simulink model "snb_bc"  (R2012b)
settings: Solver=FixedStepDiscrete  SolverMode=SingleTasking  StartTime=0.0  StopTime=10000  RelTol=1e-3
undefined symbols (not defined in the file): Down, pfb_coeff_gen_calc, Up
libraries: xbsIndex_r4 x19640, casper_library_misc x44, casper_library_delays x18, casper_library_communications x8, xps_library x3
(part 12 of 163)

== system snb_bc/gbe_status ==
  out_gbe0_linkup : Inport
  out_gbe1_linkup : Inport  Port=2
  out_gbe2_linkup : Inport  Port=3
  out_gbe3_linkup : Inport  Port=4
  assert_gbe0_linkup : xbsIndex_r4/Assert  assert_type=on  type_source=Explicitly  gui_display_data_type=Boolean  arith_type=Boolean  n_bits=1  bin_pt=0  preci_type=Single  exp_width=8  frac_width=24  assert_rate=off  rate_source=Explicitly  period=1  output_port=on  block_type=assert
  assert_gbe1_linkup : xbsIndex_r4/Assert  assert_type=on  type_source=Explicitly  gui_display_data_type=Boolean  arith_type=Boolean  n_bits=1  bin_pt=0  preci_type=Single  exp_width=8  frac_width=24  assert_rate=off  rate_source=Explicitly  period=1  output_port=on  block_type=assert
  assert_gbe2_linkup : xbsIndex_r4/Assert  assert_type=on  type_source=Explicitly  gui_display_data_type=Boolean  arith_type=Boolean  n_bits=1  bin_pt=0  preci_type=Single  exp_width=8  frac_width=24  assert_rate=off  rate_source=Explicitly  period=1  output_port=on  block_type=assert
  assert_gbe3_linkup : xbsIndex_r4/Assert  assert_type=on  type_source=Explicitly  gui_display_data_type=Boolean  arith_type=Boolean  n_bits=1  bin_pt=0  preci_type=Single  exp_width=8  frac_width=24  assert_rate=off  rate_source=Explicitly  period=1  output_port=on  block_type=assert
  cast_gw : xbsIndex_r4/Convert  gui_display_data_type=Fixed-point  arith_type=Unsigned  n_bits=32  bin_pt=0  float_type=Single  exp_bits=8  fraction_bits=24  quantization=Truncate  overflow=Wrap  en=off  latency=0  dbl_ovrd=off  pipeline=off  block_type=convert
  concatenate : xbsIndex_r4/Concat  num_inputs=4  dbl_ovrd=off  block_type=concat
  io_delay : xbsIndex_r4/Delay  rst=off  infoeditControl=Selection of Reset will increase slice count due to use of real FFs and instead of SRLs  en=off  latency=0  dbl_ovrd=off  reg_retiming=on  block_type=delay
  reint{1..4} (4 alike) : xbsIndex_r4/Reinterpret  force_arith_type=on  arith_type=Unsigned  force_bin_pt=on  bin_pt=0  block_type=reinterpret
  sim_out : Terminator
  snb_bc_gbe_status_user_data_in : xbsIndex_r4/Gateway Out  inherit_from_input=off  hdl_port=on  timing_constraint=None  locs_specified=off  LOCs={}  UseAsDAC=off  DACChannel='1'  block_type=gatewayout
  wires:
  concatenate/1 -> io_delay/1
  io_delay/1 -> cast_gw/1
  cast_gw/1 -> snb_bc_gbe_status_user_data_in/1
  snb_bc_gbe_status_user_data_in/1 -> sim_out/1
  out_gbe0_linkup/1 -> assert_gbe0_linkup/1
  assert_gbe0_linkup/1 -> reint1/1
  reint1/1 -> concatenate/1
  out_gbe1_linkup/1 -> assert_gbe1_linkup/1
  assert_gbe1_linkup/1 -> reint2/1
  reint2/1 -> concatenate/2
  out_gbe2_linkup/1 -> assert_gbe2_linkup/1
  assert_gbe2_linkup/1 -> reint3/1
  reint3/1 -> concatenate/3
  out_gbe3_linkup/1 -> assert_gbe3_linkup/1
  assert_gbe3_linkup/1 -> reint4/1
  reint4/1 -> concatenate/4

== system snb_bc/generate_pkt_sync ==
  sync : Inport
  valid : Inport  Port=2
  data : Inport  Port=3
  Constant : xbsIndex_r4/Constant  const=(2^pktlen_bits)-1  gui_display_data_type=Fixed-point  arith_type=Unsigned  n_bits=pktlen_bits  bin_pt=0  preci_type=Single  exp_width=8  frac_width=24  explicit_period=on  period=1  equ=P=C  opselect=C  inp2=PCIN>>17  opr=+  inp1=P  carry=CIN  dbl_ovrd=off  block_type=constant
  Counter1 : xbsIndex_r4/Counter  cnt_type=Free Running  cnt_to=Inf  operation=Up  start_count=0  cnt_by_val=1  arith_type=Unsigned  n_bits=pktlen_bits  bin_pt=0  load_pin=off  rst=on  en=on  explicit_period=on  period=1  dbl_ovrd=off  use_behavioral_HDL=off  implementation=Fabric  block_type=counter
  Delay : xbsIndex_r4/Delay  rst=off  infoeditControl=Selection of Reset will increase slice count due to use of real FFs and instead of SRLs  en=off  latency=1  dbl_ovrd=off  reg_retiming=off  block_type=delay
  Delay1 : xbsIndex_r4/Delay  rst=off  infoeditControl=Selection of Reset will increase slice count due to use of real FFs and instead of SRLs  en=off  latency=1  dbl_ovrd=off  reg_retiming=off  block_type=delay
  Delay2 : xbsIndex_r4/Delay  rst=off  infoeditControl=Selection of Reset will increase slice count due to use of real FFs and instead of SRLs  en=off  latency=1  dbl_ovrd=off  reg_retiming=off  block_type=delay
  Logical : xbsIndex_r4/Logical  logical_function=OR  inputs=2  en=off  latency=1  precision=Full  arith_type=Unsigned  n_bits=16  bin_pt=0  align_bp=on  dbl_ovrd=off  block_type=logical
  Logical1 : xbsIndex_r4/Logical  logical_function=AND  inputs=2  en=off  latency=0  precision=Full  arith_type=Unsigned  n_bits=16  bin_pt=0  align_bp=on  dbl_ovrd=off  block_type=logical
  Relational : xbsIndex_r4/Relational  mode=a=b  en=off  latency=0  dbl_ovrd=off  block_type=relational
  out_sync : Outport
  out_valid : Outport  Port=2
  out_data : Outport  Port=3
  packet_sync : Outport  Port=4
  wires:
  valid/1 -> Delay/1, Logical1/1, Counter1/2
  Counter1/1 -> Relational/1  "pkt_counter"
  sync/1 -> Logical/1, Delay1/1, Counter1/1
  Delay/1 -> out_valid/1
  Delay1/1 -> out_sync/1
  Delay2/1 -> out_data/1
  data/1 -> Delay2/1
  Constant/1 -> Relational/2
  Relational/1 -> Logical1/2
  Logical1/1 -> Logical/2  "ns"
  Logical/1 -> packet_sync/1

== system snb_bc/generate_pkt_sync1 ==
  sync : Inport
  valid : Inport  Port=2
  data : Inport  Port=3
  Constant : xbsIndex_r4/Constant  const=(2^pktlen_bits)-1  gui_display_data_type=Fixed-point  arith_type=Unsigned  n_bits=pktlen_bits  bin_pt=0  preci_type=Single  exp_width=8  frac_width=24  explicit_period=on  period=1  equ=P=C  opselect=C  inp2=PCIN>>17  opr=+  inp1=P  carry=CIN  dbl_ovrd=off  block_type=constant
  Counter1 : xbsIndex_r4/Counter  cnt_type=Free Running  cnt_to=Inf  operation=Up  start_count=0  cnt_by_val=1  arith_type=Unsigned  n_bits=pktlen_bits  bin_pt=0  load_pin=off  rst=on  en=on  explicit_period=on  period=1  dbl_ovrd=off  use_behavioral_HDL=off  implementation=Fabric  block_type=counter
  Delay : xbsIndex_r4/Delay  rst=off  infoeditControl=Selection of Reset will increase slice count due to use of real FFs and instead of SRLs  en=off  latency=1  dbl_ovrd=off  reg_retiming=off  block_type=delay
  Delay1 : xbsIndex_r4/Delay  rst=off  infoeditControl=Selection of Reset will increase slice count due to use of real FFs and instead of SRLs  en=off  latency=1  dbl_ovrd=off  reg_retiming=off  block_type=delay
  Delay2 : xbsIndex_r4/Delay  rst=off  infoeditControl=Selection of Reset will increase slice count due to use of real FFs and instead of SRLs  en=off  latency=1  dbl_ovrd=off  reg_retiming=off  block_type=delay
  Logical : xbsIndex_r4/Logical  logical_function=OR  inputs=2  en=off  latency=1  precision=Full  arith_type=Unsigned  n_bits=16  bin_pt=0  align_bp=on  dbl_ovrd=off  block_type=logical
  Logical1 : xbsIndex_r4/Logical  logical_function=AND  inputs=2  en=off  latency=0  precision=Full  arith_type=Unsigned  n_bits=16  bin_pt=0  align_bp=on  dbl_ovrd=off  block_type=logical
  Relational : xbsIndex_r4/Relational  mode=a=b  en=off  latency=0  dbl_ovrd=off  block_type=relational
  out_sync : Outport
  out_valid : Outport  Port=2
  out_data : Outport  Port=3
  packet_sync : Outport  Port=4
  wires:
  valid/1 -> Delay/1, Logical1/1, Counter1/2
  Counter1/1 -> Relational/1  "pkt_counter"
  sync/1 -> Logical/1, Delay1/1, Counter1/1
  Delay/1 -> out_valid/1
  Delay1/1 -> out_sync/1
  Delay2/1 -> out_data/1
  data/1 -> Delay2/1
  Constant/1 -> Relational/2
  Relational/1 -> Logical1/2
  Logical1/1 -> Logical/2  "ns"
  Logical/1 -> packet_sync/1

== system snb_bc/iptx_base ==
  sim_1 : Inport
  io_delay : xbsIndex_r4/Delay  rst=off  infoeditControl=Selection of Reset will increase slice count due to use of real FFs and instead of SRLs  en=off  latency=0  dbl_ovrd=off  reg_retiming=on  block_type=delay
  reint1 : xbsIndex_r4/Reinterpret  force_arith_type=on  arith_type=Unsigned  force_bin_pt=on  bin_pt=0  block_type=reinterpret
  slice_reg : xbsIndex_r4/Slice  nbits=32  boolean_output=off  mode=Lower Bit Location + Width  bit1=0  base1=MSB of Input  bit0=0  base0=LSB of Input  dbl_ovrd=off  block_type=slice
  snb_bc_iptx_base_user_data_out : xbsIndex_r4/Gateway In  gui_display_data_type=Fixed-point  arith_type=Unsigned  n_bits=32  bin_pt=0  preci_type=Single  exp_width=8  frac_width=24  quantization="Round  (unbiased: +/- Inf)"  overflow=Saturate  period=1  dbl_ovrd=off  timing_constraint=None  locs_specified=off  LOCs={}  UseAsADC=off  ADCChannel='1'  inherit_from_input=off  hdl_port=on  block_type=gatewayin
  in_reg : Outport
  wires:
  snb_bc_iptx_base_user_data_out/1 -> io_delay/1
  sim_1/1 -> snb_bc_iptx_base_user_data_out/1
  io_delay/1 -> slice_reg/1
  slice_reg/1 -> reint1/1
  reint1/1 -> in_reg/1

== system snb_bc/local_time_lsw ==
  out_timestamp_lsw : Inport
  assert_timestamp_lsw : xbsIndex_r4/Assert  assert_type=on  type_source=Explicitly  gui_display_data_type=Fixed-point  arith_type=Unsigned  n_bits=32  bin_pt=0  preci_type=Single  exp_width=8  frac_width=24  assert_rate=off  rate_source=Explicitly  period=1  output_port=on  block_type=assert
  cast_gw : xbsIndex_r4/Convert  gui_display_data_type=Fixed-point  arith_type=Unsigned  n_bits=32  bin_pt=0  float_type=Single  exp_bits=8  fraction_bits=24  quantization=Truncate  overflow=Wrap  en=off  latency=0  dbl_ovrd=off  pipeline=off  block_type=convert
  io_delay : xbsIndex_r4/Delay  rst=off  infoeditControl=Selection of Reset will increase slice count due to use of real FFs and instead of SRLs  en=off  latency=0  dbl_ovrd=off  reg_retiming=on  block_type=delay
  reint1 : xbsIndex_r4/Reinterpret  force_arith_type=on  arith_type=Unsigned  force_bin_pt=on  bin_pt=0  block_type=reinterpret
  sim_out : Terminator
  snb_bc_local_time_lsw_user_data_in : xbsIndex_r4/Gateway Out  inherit_from_input=off  hdl_port=on  timing_constraint=None  locs_specified=off  LOCs={}  UseAsDAC=off  DACChannel='1'  block_type=gatewayout
  wires:
  io_delay/1 -> cast_gw/1
  cast_gw/1 -> snb_bc_local_time_lsw_user_data_in/1
  snb_bc_local_time_lsw_user_data_in/1 -> sim_out/1
  out_timestamp_lsw/1 -> assert_timestamp_lsw/1
  assert_timestamp_lsw/1 -> reint1/1
  reint1/1 -> io_delay/1

== system snb_bc/local_time_msw ==
  out_timestamp_msw : Inport
  assert_timestamp_msw : xbsIndex_r4/Assert  assert_type=on  type_source=Explicitly  gui_display_data_type=Fixed-point  arith_type=Unsigned  n_bits=32  bin_pt=0  preci_type=Single  exp_width=8  frac_width=24  assert_rate=off  rate_source=Explicitly  period=1  output_port=on  block_type=assert
  cast_gw : xbsIndex_r4/Convert  gui_display_data_type=Fixed-point  arith_type=Unsigned  n_bits=32  bin_pt=0  float_type=Single  exp_bits=8  fraction_bits=24  quantization=Truncate  overflow=Wrap  en=off  latency=0  dbl_ovrd=off  pipeline=off  block_type=convert
  io_delay : xbsIndex_r4/Delay  rst=off  infoeditControl=Selection of Reset will increase slice count due to use of real FFs and instead of SRLs  en=off  latency=0  dbl_ovrd=off  reg_retiming=on  block_type=delay
  reint1 : xbsIndex_r4/Reinterpret  force_arith_type=on  arith_type=Unsigned  force_bin_pt=on  bin_pt=0  block_type=reinterpret
  sim_out : Terminator
  snb_bc_local_time_msw_user_data_in : xbsIndex_r4/Gateway Out  inherit_from_input=off  hdl_port=on  timing_constraint=None  locs_specified=off  LOCs={}  UseAsDAC=off  DACChannel='1'  block_type=gatewayout
  wires:
  io_delay/1 -> cast_gw/1
  cast_gw/1 -> snb_bc_local_time_msw_user_data_in/1
  snb_bc_local_time_msw_user_data_in/1 -> sim_out/1
  out_timestamp_msw/1 -> assert_timestamp_msw/1
  assert_timestamp_msw/1 -> reint1/1
  reint1/1 -> io_delay/1

== system snb_bc/mcnt_relock ==
  out_reg : Inport
  assert_reg : xbsIndex_r4/Assert  assert_type=on  type_source=Explicitly  gui_display_data_type=Fixed-point  arith_type=Unsigned  n_bits=32  bin_pt=0  preci_type=Single  exp_width=8  frac_width=24  assert_rate=off  rate_source=Explicitly  period=1  output_port=on  block_type=assert
  cast_gw : xbsIndex_r4/Convert  gui_display_data_type=Fixed-point  arith_type=Unsigned  n_bits=32  bin_pt=0  float_type=Single  exp_bits=8  fraction_bits=24  quantization=Truncate  overflow=Wrap  en=off  latency=0  dbl_ovrd=off  pipeline=off  block_type=convert
  io_delay : xbsIndex_r4/Delay  rst=off  infoeditControl=Selection of Reset will increase slice count due to use of real FFs and instead of SRLs  en=off  latency=0  dbl_ovrd=off  reg_retiming=on  block_type=delay
  reint1 : xbsIndex_r4/Reinterpret  force_arith_type=on  arith_type=Unsigned  force_bin_pt=on  bin_pt=0  block_type=reinterpret
  sim_out : Terminator
  snb_bc_mcnt_relock_user_data_in : xbsIndex_r4/Gateway Out  inherit_from_input=off  hdl_port=on  timing_constraint=None  locs_specified=off  LOCs={}  UseAsDAC=off  DACChannel='1'  block_type=gatewayout
  wires:
  io_delay/1 -> cast_gw/1
  cast_gw/1 -> snb_bc_mcnt_relock_user_data_in/1
  snb_bc_mcnt_relock_user_data_in/1 -> sim_out/1
  out_reg/1 -> assert_reg/1
  assert_reg/1 -> reint1/1
  reint1/1 -> io_delay/1

== system snb_bc/mix_dec_fir ==
  note: f20.18 output
  note: 4/16 = (1712 * 4/16) = 428Mhz
  dvin : Inport
  syncin : Inport  Port=2
  pol0 : Inport  Port=3
  pol1 : Inport  Port=4
  Convert{,1..31} (32 alike) : xbsIndex_r4/Convert  gui_display_data_type=Fixed-point  arith_type="Signed  (2's comp)"  n_bits=10  bin_pt=9  float_type=Single  exp_bits=8  fraction_bits=24  quantization=Truncate  overflow=Wrap  en=off  latency=0  dbl_ovrd=off  pipeline=off  block_type=convert
  Delay : xbsIndex_r4/Delay  rst=off  infoeditControl=Selection of Reset will increase slice count due to use of real FFs and instead of SRLs  en=off  latency=4  dbl_ovrd=off  reg_retiming=off  block_type=delay
  Terminator1 : Terminator
  Terminator11 : Terminator
  bus_create : Subsystem  AncestorBlock=casper_library_flow_control/bus_create  mask(bus_create){inputNum=16}
      mask prompts: inputNum "Number of inputs:"
      mask init:
      | bus_create_init(gcb,...
      |     'inputNum', inputNum);
  bus_create1 : Subsystem  AncestorBlock=casper_library_flow_control/bus_create  mask(bus_create){inputNum=16}
      mask prompts: inputNum "Number of inputs:"
      mask init:
      | bus_create_init(gcb,...
      |     'inputNum', inputNum);
  bus_expand16 : Subsystem  AncestorBlock=casper_library_flow_control/bus_expand  mask(bus_expand){mode=divisions of equal size, outputNum=8, outputWidth=10, outputBinaryPt=9, outputArithmeticType=1, show_format=off, outputToWorkspace=off, variablePrefix=out, outputToModelAsWell=on}
      mask prompts: outputNum "Number of outputs:"; outputWidth "Output width:"; outputBinaryPt "Output binary point position:"; outputArithmeticType "Output arithmetic type (ufix=0, fix=1, bool=2):"; show_format "Print format string?"; outputToWorkspace "Output to workspace?"; variablePrefix "Variable name prefix:"; outputToModelAsWell "Output to model as well?"
      mask help:
      | Expands a 'bus' made using a bus_create or Xilinx
      | concat block.
      | The input will be divided into the specified number
      | of outputs with the specified arithmetic types.
      | Divisions are made from most significant bit.
      mask init: same as snb_bc/bus_expand10
      settings: AttributesFormatString=8 outputs
      mask TypeOptions mode: divisions of equal size | divisions of arbitrary size
      mask Callback mode: bus_expand_callback();
      mask Callback outputWidth: bus_expand_callback();
      mask Callback outputToWorkspace: bus_expand_callback();
  bus_expand17 : Subsystem  AncestorBlock=casper_library_flow_control/bus_expand  mask(bus_expand){mode=divisions of equal size, outputNum=8, outputWidth=10, outputBinaryPt=9, outputArithmeticType=1, show_format=off, outputToWorkspace=off, variablePrefix=out, outputToModelAsWell=on}
      mask prompts: outputNum "Number of outputs:"; outputWidth "Output width:"; outputBinaryPt "Output binary point position:"; outputArithmeticType "Output arithmetic type (ufix=0, fix=1, bool=2):"; show_format "Print format string?"; outputToWorkspace "Output to workspace?"; variablePrefix "Variable name prefix:"; outputToModelAsWell "Output to model as well?"
      mask help:
      | Expands a 'bus' made using a bus_create or Xilinx
      | concat block.
      | The input will be divided into the specified number
      | of outputs with the specified arithmetic types.
      | Divisions are made from most significant bit.
      mask init: same as snb_bc/bus_expand10
      settings: AttributesFormatString=8 outputs
      mask TypeOptions mode: divisions of equal size | divisions of arbitrary size
      mask Callback mode: bus_expand_callback();
      mask Callback outputWidth: bus_expand_callback();
      mask Callback outputToWorkspace: bus_expand_callback();
  dec_fir_async : Subsystem  Tag=casper:dec_fir_async  AncestorBlock=casper_library_downconverter/dec_fir_async  mask(dec_fir_async){n_inputs=8, coeff=|, output_width=18, output_bp=17, quantization=Round  (unbiased: +/- Inf), add_latency=5, mult_latency=5, conv_latency=5, coeff_bit_width=24, coeff_bin_pt=23, lshift=0, absorb_adders=off, adder_imp=Behavioral, async=on, bus_input=on, input_width=10, input_bp=9, input_type=Signed}
      mask coeff=|
      | [-0.000270647030267098	-0.000122723037134337	-8.23265588475279e-05	3.75975512915862e-06	0.000150550359161717	0.000374548378332765	0.000693303775510887	0.00112485015838604	0.00168703305075908	0.00239674972617759	0.00326912752959290	0.00431667355778343	0.00554843321823961	0.00696919817534850	0.00857880523379181	0.0103715666112793	0.0123358687396821	0.0144539712538508	0.0167020303575575	0.0190503615961945	0.0214639466270833	0.0239031773625389	0.0263248194350674	0.0286831658989276	0.0309313420381547	0.0330227136630624	0.0349123448410226	0.0365584470190412	0.0379237602263779	0.0389768086231192	0.0396929770598783	0.0400553623551974	0.0400553623551974	0.0396929770598783	0.0389768086231192	0.0379237602263779	0.0365584470190412	0.0349123448410226	0.0330227136630624	0.0309313420381547	0.0286831658989276	0.0263248194350674	0.0239031773625389	0.0214639466270833	0.0190503615961945	0.0167020303575575	0.0144539712538508	0.0123358687396821	0.0103715666112793	0.00857880523379181	0.00696919817534850	0.00554843321823961	0.00431667355778343	0.00326912752959290	0.00239674972617759	0.00168703305075908	0.00112485015838604	0.000693303775510887	0.000374548378332765	0.000150550359161717	3.75975512915862e-06	-8.23265588475279e-05	-0.000122723037134337	-0.000270647030267098
      | ]
      mask prompts: n_inputs "Number of Parallel Streams"; coeff "Coefficients"; output_width "Output bitwidth"; output_bp "Output binary point"; quantization "Quantization Behavior"; add_latency "Add Latency"; mult_latency "Mult Latency"; conv_latency "Convert latency"; coeff_bit_width "Coefficient bitwidth"; coeff_bin_pt "Coefficient binary point"; lshift "Post adder-tree shift"; absorb_adders "Absorb adders into DSP slices"; adder_imp "Adder implementation"; async "Asynchronous ops"; bus_input "Bus input"; input_width "Input bitwidth"; input_bp "Input binary point"; input_type "Input datatype"
      mask help: FIR filter which can handle multiple time samples in parallel and decimates down to 1 time sample. If coefficients are symmetric, will automatically fold before multiplying.
      mask init:
      | dec_fir_async_init(gcb);
      settings: AttributesFormatString=|
      | 64 taps
      | 18_17 r/i
      mask TypeOptions quantization: Truncate | Round  (unbiased: +/- Inf) | Round  (unbiased: Even Values)
      mask TypeOptions adder_imp: Behavioral | Fabric | DSP48
      mask Callback bus_input:
      | onoff = get_param(gcb, 'bus_input');
      | set_param_state(gcb, 'input_width', onoff)
      | set_param_state(gcb, 'input_bp', onoff)
      | set_param_state(gcb, 'input_type', onoff)
      mask TypeOptions input_type: Signed | Unsigned
  dec_fir_async1 : Subsystem  Tag=casper:dec_fir_async  AncestorBlock=casper_library_downconverter/dec_fir_async  mask(dec_fir_async){n_inputs=8, coeff=|, output_width=18, output_bp=17, quantization=Round  (unbiased: +/- Inf), add_latency=5, mult_latency=5, conv_latency=5, coeff_bit_width=24, coeff_bin_pt=23, lshift=0, absorb_adders=off, adder_imp=Behavioral, async=on, bus_input=on, input_width=10, input_bp=9, input_type=Signed}
      mask coeff=|
      | [-0.000270647030267098	-0.000122723037134337	-8.23265588475279e-05	3.75975512915862e-06	0.000150550359161717	0.000374548378332765	0.000693303775510887	0.00112485015838604	0.00168703305075908	0.00239674972617759	0.00326912752959290	0.00431667355778343	0.00554843321823961	0.00696919817534850	0.00857880523379181	0.0103715666112793	0.0123358687396821	0.0144539712538508	0.0167020303575575	0.0190503615961945	0.0214639466270833	0.0239031773625389	0.0263248194350674	0.0286831658989276	0.0309313420381547	0.0330227136630624	0.0349123448410226	0.0365584470190412	0.0379237602263779	0.0389768086231192	0.0396929770598783	0.0400553623551974	0.0400553623551974	0.0396929770598783	0.0389768086231192	0.0379237602263779	0.0365584470190412	0.0349123448410226	0.0330227136630624	0.0309313420381547	0.0286831658989276	0.0263248194350674	0.0239031773625389	0.0214639466270833	0.0190503615961945	0.0167020303575575	0.0144539712538508	0.0123358687396821	0.0103715666112793	0.00857880523379181	0.00696919817534850	0.00554843321823961	0.00431667355778343	0.00326912752959290	0.00239674972617759	0.00168703305075908	0.00112485015838604	0.000693303775510887	0.000374548378332765	0.000150550359161717	3.75975512915862e-06	-8.23265588475279e-05	-0.000122723037134337	-0.000270647030267098
      | ]
      mask prompts: n_inputs "Number of Parallel Streams"; coeff "Coefficients"; output_width "Output bitwidth"; output_bp "Output binary point"; quantization "Quantization Behavior"; add_latency "Add Latency"; mult_latency "Mult Latency"; conv_latency "Convert latency"; coeff_bit_width "Coefficient bitwidth"; coeff_bin_pt "Coefficient binary point"; lshift "Post adder-tree shift"; absorb_adders "Absorb adders into DSP slices"; adder_imp "Adder implementation"; async "Asynchronous ops"; bus_input "Bus input"; input_width "Input bitwidth"; input_bp "Input binary point"; input_type "Input datatype"
      mask help: FIR filter which can handle multiple time samples in parallel and decimates down to 1 time sample. If coefficients are symmetric, will automatically fold before multiplying.
      mask init:
      | dec_fir_async_init(gcb);
      settings: AttributesFormatString=|
      | 64 taps
      | 18_17 r/i
      mask TypeOptions quantization: Truncate | Round  (unbiased: +/- Inf) | Round  (unbiased: Even Values)
      mask TypeOptions adder_imp: Behavioral | Fabric | DSP48
      mask Callback bus_input:
      | onoff = get_param(gcb, 'bus_input');
      | set_param_state(gcb, 'input_width', onoff)
      | set_param_state(gcb, 'input_bp', onoff)
      | set_param_state(gcb, 'input_type', onoff)
      mask TypeOptions input_type: Signed | Unsigned
  mixer : Subsystem  Tag=casper:mixer  AncestorBlock=casper_library_downconverter/mixer  mask(mixer){freq_div=16, freq=4, nstreams=8, n_bits=10, bram_latency=2, mult_latency=4}
      mask prompts: freq_div "Frequency Divisions (M)"; freq "Mixing Frequency (? / M*2pi)"; nstreams "Number of Parallel Streams"; n_bits "Bit Width"; bram_latency "BRAM Latency"; mult_latency "Mult Latency"
      mask help: Digitally mixes an input signal (which can be several samples in parallel) with an LO of the indicated frequency (which is some fraction of the native FPGA clock rate).
      mask init:
      | mixer_init(gcb, ...
      |     'freq_div', freq_div, ...
      |     'freq', freq, ...
      |     'nstreams', nstreams, ...
      |     'n_bits', n_bits, ...
      |     'bram_latency', bram_latency, ...
      |     'mult_latency', mult_latency);
      settings: AttributesFormatString=lo at -4/16
  mixer1 : Subsystem  Tag=casper:mixer  AncestorBlock=casper_library_downconverter/mixer  mask(mixer){freq_div=16, freq=4, nstreams=8, n_bits=10, bram_latency=2, mult_latency=4}
      mask prompts: freq_div "Frequency Divisions (M)"; freq "Mixing Frequency (? / M*2pi)"; nstreams "Number of Parallel Streams"; n_bits "Bit Width"; bram_latency "BRAM Latency"; mult_latency "Mult Latency"
      mask help: Digitally mixes an input signal (which can be several samples in parallel) with an LO of the indicated frequency (which is some fraction of the native FPGA clock rate).
      mask init: same as snb_bc/mix_dec_fir/mixer
      settings: AttributesFormatString=lo at -4/16
  pipeline1 : Subsystem  AncestorBlock=casper_library_delays/pipeline  mask(pipeline){latency=3}
      mask help:
      | An explicitly laid-out delay line to avoid mapping to SRL16s
      | for use in pipelining to help achieve timing closure.
      mask init:
      | pipeline_init(gcb,'latency',latency);
      settings: AttributesFormatString=Latency = %<latency>
      mask Display:
      | port_label('input', 1, 'd');
      | port_label('output', 1, 'q');
      | disp(['Z^-', num2str(latency)]);
  pipeline2 : Subsystem  AncestorBlock=casper_library_delays/pipeline  mask(pipeline){latency=3}
      mask help:
      | An explicitly laid-out delay line to avoid mapping to SRL16s
      | for use in pipelining to help achieve timing closure.
      mask init:
      | pipeline_init(gcb,'latency',latency);
      settings: AttributesFormatString=Latency = %<latency>
      mask Display:
      | port_label('input', 1, 'd');
      | port_label('output', 1, 'q');
      | disp(['Z^-', num2str(latency)]);
  pipeline29 : Subsystem  AncestorBlock=casper_library_delays/pipeline  mask(pipeline){latency=3}
      mask help:
      | An explicitly laid-out delay line to avoid mapping to SRL16s
      | for use in pipelining to help achieve timing closure.
      mask init:
      | pipeline_init(gcb,'latency',latency);
      settings: AttributesFormatString=Latency = %<latency>
      mask Display:
      | port_label('input', 1, 'd');
      | port_label('output', 1, 'q');
      | disp(['Z^-', num2str(latency)]);
  pipeline3 : Subsystem  AncestorBlock=casper_library_delays/pipeline  mask(pipeline){latency=3}
      mask help:
      | An explicitly laid-out delay line to avoid mapping to SRL16s
      | for use in pipelining to help achieve timing closure.
      mask init:
      | pipeline_init(gcb,'latency',latency);
      settings: AttributesFormatString=Latency = %<latency>
      mask Display:
      | port_label('input', 1, 'd');
      | port_label('output', 1, 'q');
      | disp(['Z^-', num2str(latency)]);
  pipeline4 : Subsystem  AncestorBlock=casper_library_delays/pipeline  mask(pipeline){latency=3}
      mask help:
      | An explicitly laid-out delay line to avoid mapping to SRL16s
      | for use in pipelining to help achieve timing closure.
      mask init:
      | pipeline_init(gcb,'latency',latency);
      settings: AttributesFormatString=Latency = %<latency>
      mask Display:
      | port_label('input', 1, 'd');
      | port_label('output', 1, 'q');
      | disp(['Z^-', num2str(latency)]);
  pipeline5 : Subsystem  AncestorBlock=casper_library_delays/pipeline  mask(pipeline){latency=3}
      mask help:
      | An explicitly laid-out delay line to avoid mapping to SRL16s
      | for use in pipelining to help achieve timing closure.
      mask init:
      | pipeline_init(gcb,'latency',latency);
      settings: AttributesFormatString=Latency = %<latency>
      mask Display:
      | port_label('input', 1, 'd');
      | port_label('output', 1, 'q');
      | disp(['Z^-', num2str(latency)]);
  sync_out : Outport
  pol0_out : Outport  Port=2
  pol1_out : Outport  Port=3
  dv_out : Outport  Port=4
  wires:
  mixer/1(sync_out) -> pipeline29/1(d)
  mixer/2(real1) -> Convert/1
  mixer/6(real3) -> Convert5/1
  mixer/3(imag1) -> Convert2/1
  mixer/4(real2) -> Convert3/1
  mixer/7(imag3) -> Convert6/1
  mixer/10(real5) -> Convert9/1
  mixer/12(real6) -> Convert13/1
  mixer/8(real4) -> Convert7/1
  mixer/16(real8) -> Convert16/1
  mixer/11(imag5) -> Convert10/1
  mixer/14(real7) -> Convert15/1
  mixer/13(imag6) -> Convert14/1
  mixer/15(imag7) -> Convert11/1
  mixer/17(imag8) -> Convert12/1
  mixer/9(imag4) -> Convert8/1
  mixer/5(imag2) -> Convert4/1
  syncin/1 -> mixer1/1(sync), mixer/1(sync)
  bus_create/1(bus_out) -> pipeline2/1(d)
  dvin/1 -> Delay/1
  Delay/1 -> pipeline4/1(d), pipeline1/1(d)
  bus_expand17/5(out4) -> mixer/6(din5)
  bus_expand17/2(out7) -> mixer/3(din2)
  bus_expand17/4(out5) -> mixer/5(din4)
  bus_expand17/3(out6) -> mixer/4(din3)
  bus_expand17/7(out2) -> mixer/8(din7)
  bus_expand17/6(out3) -> mixer/7(din6)
  bus_expand17/1(msb_out8) -> mixer/2(din1)
  bus_expand17/8(lsb_out1) -> mixer/9(din8)
  pol0/1 -> bus_expand17/1(bus_in)
  dec_fir_async/1(sync_out) -> sync_out/1
  dec_fir_async/2(dout) -> pol0_out/1
  dec_fir_async/3(dv_out) -> dv_out/1
  mixer1/1(sync_out) -> pipeline3/1(d)
  mixer1/2(real1) -> Convert1/1
  mixer1/6(real3) -> Convert27/1
  mixer1/3(imag1) -> Convert24/1
  mixer1/4(real2) -> Convert25/1
  mixer1/7(imag3) -> Convert28/1
  mixer1/10(real5) -> Convert31/1
  mixer1/12(real6) -> Convert20/1
  mixer1/8(real4) -> Convert29/1
  mixer1/16(real8) -> Convert23/1
  mixer1/11(imag5) -> Convert17/1
  mixer1/14(real7) -> Convert22/1
  mixer1/13(imag6) -> Convert21/1
  mixer1/15(imag7) -> Convert18/1
  mixer1/17(imag8) -> Convert19/1
  mixer1/9(imag4) -> Convert30/1
  mixer1/5(imag2) -> Convert26/1
  bus_create1/1(bus_out) -> pipeline5/1(d)
  bus_expand16/5(out4) -> mixer1/6(din5)
  bus_expand16/2(out7) -> mixer1/3(din2)
  bus_expand16/4(out5) -> mixer1/5(din4)
  bus_expand16/3(out6) -> mixer1/4(din3)
  bus_expand16/7(out2) -> mixer1/8(din7)
  bus_expand16/6(out3) -> mixer1/7(din6)
  bus_expand16/1(msb_out8) -> mixer1/2(din1)
  bus_expand16/8(lsb_out1) -> mixer1/9(din8)
  pol1/1 -> bus_expand16/1(bus_in)
  dec_fir_async1/1(sync_out) -> Terminator11/1
  dec_fir_async1/2(dout) -> pol1_out/1
  dec_fir_async1/3(dv_out) -> Terminator1/1
  pipeline29/1(q) -> dec_fir_async/1(sync_in)
  pipeline1/1(q) -> dec_fir_async/2(dv_in)
  pipeline2/1(q) -> dec_fir_async/3(dbus_in)
  pipeline3/1(q) -> dec_fir_async1/1(sync_in)
  pipeline4/1(q) -> dec_fir_async1/2(dv_in)
  pipeline5/1(q) -> dec_fir_async1/3(dbus_in)
  Convert29/1 -> bus_create1/7(in7)
  Convert20/1 -> bus_create1/11(in11)
  Convert17/1 -> bus_create1/10(in10)
  Convert1/1 -> bus_create1/1(in1)
  Convert25/1 -> bus_create1/3(in3)
  Convert31/1 -> bus_create1/9(in9)
  Convert19/1 -> bus_create1/16(in16)
  Convert26/1 -> bus_create1/4(in4)
  Convert22/1 -> bus_create1/13(in13)
  Convert27/1 -> bus_create1/5(in5)
  Convert28/1 -> bus_create1/6(in6)
  Convert30/1 -> bus_create1/8(in8)
  Convert21/1 -> bus_create1/12(in12)
  Convert24/1 -> bus_create1/2(in2)
  Convert18/1 -> bus_create1/14(in14)
  Convert23/1 -> bus_create1/15(in15)
  Convert12/1 -> bus_create/16(in16)
  Convert16/1 -> bus_create/15(in15)
  Convert14/1 -> bus_create/12(in12)
  Convert8/1 -> bus_create/8(in8)
  Convert3/1 -> bus_create/3(in3)
  Convert/1 -> bus_create/1(in1)
  Convert15/1 -> bus_create/13(in13)
  Convert6/1 -> bus_create/6(in6)
  Convert13/1 -> bus_create/11(in11)
  Convert9/1 -> bus_create/9(in9)
  Convert7/1 -> bus_create/7(in7)
  Convert5/1 -> bus_create/5(in5)
  Convert2/1 -> bus_create/2(in2)
  Convert11/1 -> bus_create/14(in14)
  Convert4/1 -> bus_create/4(in4)
  Convert10/1 -> bus_create/10(in10)

== system snb_bc/oneshot ==
  arm : Inport
  trigger : Inport  Port=2
  Logical1 : xbsIndex_r4/Logical  logical_function=AND  inputs=2  en=off  latency=0  precision=Full  arith_type=Unsigned  n_bits=16  bin_pt=0  align_bp=on  dbl_ovrd=off  block_type=logical
  Register1 : xbsIndex_r4/Register  init=0  rst=on  en=on  dbl_ovrd=off  block_type=register
  edge_detect1 : Subsystem  AncestorBlock=casper_library_misc/edge_detect  mask(edge_detect){edge=Rising, polarity=Active High, x_in=[0 0.08 0.08 0.16 0.16 0.24 0.24 0.32 0.32 0.4], y_in=[-1 -1  1  1  1  1  1  1  1  1], x_out=[0.6 0.68 0.68 0.76 0.76 0.84 0.84 0.92 0.92 1], y_out=[-1 -1  1  1 -1 -1 -1 -1 -1 -1]}
      mask prompts: edge "Edge Type"; polarity "Output Polarity"; x_in "Input X Positions"; y_in "Input Y Positions"; x_out "Output X Positions"; y_out "Output Y Positions"
      mask help: Output is active for one-cycle after each edge of the specified type (i.e. rising, falling or both).
      mask init: same as snb_bc/edge_detect1
      settings: AttributesFormatString=|
      | rising edges
      | active high
      mask Help: Output is active for one-cycle after each edge of the specified type (i.e. rising, falling, or both).  Latency is zero.
      mask TypeOptions edge: Rising | Falling | Both
      mask TypeOptions polarity: Active High | Active Low
      mask Display:
      | plot(x_in_num,0.5+y_in_num*0.2);
      | plot(x_out_num,0.5+y_out_num*0.2);
  oneshot : Outport
  wires:
  edge_detect1/1(out) -> Register1/3, Register1/1
  trigger/1 -> Logical1/2
  Register1/1 -> Logical1/1  "armed"
  Logical1/1 -> oneshot/1, Register1/2  "fire"
  arm/1 -> edge_detect1/1(in)

== system snb_bc/oneshot1 ==
  arm : Inport
  trigger : Inport  Port=2
  Logical1 : xbsIndex_r4/Logical  logical_function=AND  inputs=2  en=off  latency=0  precision=Full  arith_type=Unsigned  n_bits=16  bin_pt=0  align_bp=on  dbl_ovrd=off  block_type=logical
  Register1 : xbsIndex_r4/Register  init=0  rst=on  en=on  dbl_ovrd=off  block_type=register
  edge_detect1 : Subsystem  AncestorBlock=casper_library_misc/edge_detect  mask(edge_detect){edge=Rising, polarity=Active High, x_in=[0 0.08 0.08 0.16 0.16 0.24 0.24 0.32 0.32 0.4], y_in=[-1 -1  1  1  1  1  1  1  1  1], x_out=[0.6 0.68 0.68 0.76 0.76 0.84 0.84 0.92 0.92 1], y_out=[-1 -1  1  1 -1 -1 -1 -1 -1 -1]}
      mask prompts: edge "Edge Type"; polarity "Output Polarity"; x_in "Input X Positions"; y_in "Input Y Positions"; x_out "Output X Positions"; y_out "Output Y Positions"
      mask help: Output is active for one-cycle after each edge of the specified type (i.e. rising, falling or both).
      mask init: same as snb_bc/edge_detect1
      settings: AttributesFormatString=|
      | rising edges
      | active high
      mask Help: Output is active for one-cycle after each edge of the specified type (i.e. rising, falling, or both).  Latency is zero.
      mask TypeOptions edge: Rising | Falling | Both
      mask TypeOptions polarity: Active High | Active Low
      mask Display:
      | plot(x_in_num,0.5+y_in_num*0.2);
      | plot(x_out_num,0.5+y_out_num*0.2);
  oneshot : Outport
  wires:
  arm/1 -> edge_detect1/1(in)
  Logical1/1 -> Register1/2, oneshot/1  "fire"
  Register1/1 -> Logical1/1  "armed"
  trigger/1 -> Logical1/2
  edge_detect1/1(out) -> Register1/1, Register1/3

== system snb_bc/oneshot2 ==
  arm : Inport
  trigger : Inport  Port=2
  Logical1 : xbsIndex_r4/Logical  logical_function=AND  inputs=2  en=off  latency=0  precision=Full  arith_type=Unsigned  n_bits=16  bin_pt=0  align_bp=on  dbl_ovrd=off  block_type=logical
  Register1 : xbsIndex_r4/Register  init=0  rst=on  en=on  dbl_ovrd=off  block_type=register
  edge_detect1 : Subsystem  AncestorBlock=casper_library_misc/edge_detect  mask(edge_detect){edge=Rising, polarity=Active High, x_in=[0 0.08 0.08 0.16 0.16 0.24 0.24 0.32 0.32 0.4], y_in=[-1 -1  1  1  1  1  1  1  1  1], x_out=[0.6 0.68 0.68 0.76 0.76 0.84 0.84 0.92 0.92 1], y_out=[-1 -1  1  1 -1 -1 -1 -1 -1 -1]}
      mask prompts: edge "Edge Type"; polarity "Output Polarity"; x_in "Input X Positions"; y_in "Input Y Positions"; x_out "Output X Positions"; y_out "Output Y Positions"
      mask help: Output is active for one-cycle after each edge of the specified type (i.e. rising, falling or both).
      mask init: same as snb_bc/edge_detect1
      settings: AttributesFormatString=|
      | rising edges
      | active high
      mask Help: Output is active for one-cycle after each edge of the specified type (i.e. rising, falling, or both).  Latency is zero.
      mask TypeOptions edge: Rising | Falling | Both
      mask TypeOptions polarity: Active High | Active Low
      mask Display:
      | plot(x_in_num,0.5+y_in_num*0.2);
      | plot(x_out_num,0.5+y_out_num*0.2);
  oneshot : Outport
  wires:
  edge_detect1/1(out) -> Register1/3, Register1/1
  trigger/1 -> Logical1/2
  Register1/1 -> Logical1/1  "armed"
  Logical1/1 -> oneshot/1, Register1/2  "fire"
  arm/1 -> edge_detect1/1(in)
